simulink model "sensor_model"  (R2015b)
settings: Solver=VariableStepAuto  StartTime=0.0  StopTime=10.0  RelTol=1e-3
libraries: fl_lib x6, elec_lib x2, nesl_utility x2, powerlib x1
settings Model: Creator=Bastli  LastModifiedBy=Bastli

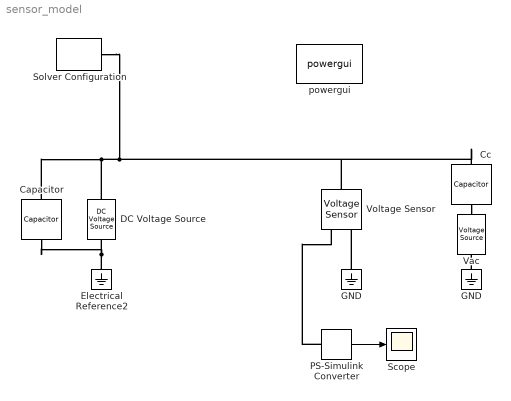
== system sensor_model ==
  Capacitor : fl_lib/Electrical/Electrical Elements/Capacitor  c=1e-6 F  r=1e-6 Ohm  g=0 1/Ohm  i_specify=off  i_priority=None  i=0 A  v_specify=off  v_priority=None  v=0 V  vc_specify=off  vc_priority=None  vc=0 V
  Cc : fl_lib/Electrical/Electrical Elements/Capacitor  c=1e-6 F  r=1e-6 Ohm  g=0 1/Ohm  i_specify=off  i_priority=None  i=0 A  v_specify=off  v_priority=None  v=0 V  vc_specify=off  vc_priority=None  vc=0 V
  DC Voltage Source : elec_lib/Additional Components/SPICE-Compatible Components/Sources/DC Voltage Source  DC=60 V
  Electrical Reference2 : fl_lib/Electrical/Electrical Elements/Electrical Reference
  GND : fl_lib/Electrical/Electrical Elements/Electrical Reference
  "GND " : fl_lib/Electrical/Electrical Elements/Electrical Reference
  PS-Simulink Converter : nesl_utility/PS-Simulink Converter  PhysicalDomain=network_engine_domain  SubClassName=ps_output  LeftPortType=input  RightPortType=output  PseudoPeriodic=off  Frequencies=[]  Unit=1  AffineConversion=off
  Scope : Scope
  Solver Configuration : nesl_utility/Solver Configuration  PhysicalDomain=network_engine_domain  SubClassName=solver  LeftPortType=input  RightPortType=generic  Accelerate=off  Tones=[]  Harmonics=[]  SimulateNoise=off  Profile=off  UseLocalSampling=off  EnableSwitchedLinearOptims=on  FrequencyDomain=off  UseCCode=off  RelTol=0.001  AbsTol=1e-06  MinStep=1e-09  ToWorkspace=off  RevertToSquareIcSolve=off  NumHomotopyIterations=100  PhasorMode=off  PhasorModeNumHarmonics=1  DoDC=on  ResidualTolerance=1e-09  UseLocalSolver=off  LocalSolverChoice=NE_BACKWARD_EULER_ADVANCER  LocalSolverSampleTime=0.001  DoFixedCost=off  MaxNonlinIter=3  MaxModeIter=2  LinearAlgebra=Sparse  DelaysMemoryBudget=1024  AutomaticFiltering=on  FilteringTimeConstant=0.001
  Vac : elec_lib/Sources/Voltage Source  dc_voltage=0 V  ac_voltage=3 V  ac_shift=0 deg  ac_frequency=60 kHz  noise_mode=0  PSD=0 V^2/Hz  sample_time=0.001 s  repeatability=1  auto_seed=3032444857  user_seed=0
  Voltage Sensor : fl_lib/Electrical/Electrical Sensors/Voltage Sensor
  powergui : powerlib/powergui  Priority=1  SimulationMode=Continuous  SolverType=Tustin/Backward Euler (TBE)  SampleTime=50e-6  frequency=60  SPID=off  DisableSnubberDevices=off  DisableRonSwitches=off  DisableVfSwitches=off  SwTol=0  DisplayEquations=off  Interpol=off  ExternalGateDelay=off  methode=off  Ts=10  FunctionMessages=off  echomessages=off  HookPort=off  EnableUseOfTLC=off  x0status=blocks  frequencyindice=60  Pbase=100e6  ErrMax=1e-4  Iterations=50  UnitsV=kV  UnitsW=MW  buscounter=0  RestoreLinks=warning  ResistiveCurrentMeasurement=off  Frange=[0:2:500]  Ylog=off  Xlog=on  ShowGrid=off  save=off  variable=ZData  structure=0  ZoomFFT=off  StartTime=0.0  cycles=1  DisplayStyle=1  fundamental=60  FreqAxis=off  MaxFrequency=1000  frequencyindicesteady=1  RmsSteady=1  display=off
  wires:
  PS-Simulink Converter/1 -> Scope/1
  connections:
  Cc/RConn1 -- Vac/LConn1
  "GND "/LConn1 -- Vac/RConn1
  GND/LConn1 -- Voltage Sensor/RConn2
  PS-Simulink Converter/LConn1 -- Voltage Sensor/RConn1
  Capacitor/RConn1 -- Electrical Reference2/LConn1 -- DC Voltage Source/RConn1
  Capacitor/LConn1 -- Cc/LConn1 -- Voltage Sensor/LConn1 -- Solver Configuration/RConn1 -- DC Voltage Source/LConn1
